simulink model "MIL4L3_SW6_V1_20220211"  (R2018b)
settings: Solver=FixedStepAuto  StartTime=0.0  StopTime=inf  FixedStep=0.001  RelTol=1e-3
PreLoadFcn:
  | A0_MILtest;
undefined symbols (not defined in the file or in its folder): Clb_ICADirect_LaneDisp_StateFive, Clb_ICADirect_LaneDisp_StateFour, Clb_ICADirect_LaneDisp_StateOne, Clb_ICADirect_LaneDisp_StateThree, Clb_ICADirect_LaneDisp_StateTwo, Clb_ICADirect_LaneDisp_StateZero, Clb_ICADirect_LaneDispSW, Clb_ICADirect_TrnLghtsCom_Switch, Clb_ICADirect_TrnLghtsCom_Value, Clb_ICADirect_TrnLghtsCrtl_Inhb, IMAP_Clb_ACU_Driver_Belt, IMAP_Clb_ACU_Driver_Belt_Over, IMAP_Clb_ACU_Passenger_Belt, IMAP_Clb_ACU_Passenger_Belt_Over, IMAP_Clb_ACU_RearLeft_Belt, IMAP_Clb_ACU_RearLeft_Belt_Over, IMAP_Clb_ACU_RearMiddle_Belt, IMAP_Clb_ACU_RearMiddle_Belt_Over, IMAP_Clb_ACU_RearRight_Belt, IMAP_Clb_ACU_RearRight_Belt_Over, IMAP_Clb_AEB_Switch, IMAP_Clb_AEB_Switch_Over, IMAP_Clb_ALC_TLC_Mode, IMAP_Clb_ALC_TLC_Mode_Over, IMAP_Clb_BCM_Battery_Voltage, IMAP_Clb_BCM_Battery_Voltage_Over, IMAP_Clb_BCM_BrakeLamp_State, IMAP_Clb_BCM_BrakeLamp_State_Over, IMAP_Clb_BCM_CHMSL_Status, IMAP_Clb_BCM_CHMSL_Status_Over, IMAP_Clb_BCM_Door_Lock_State, IMAP_Clb_BCM_Door_Lock_State_Over, IMAP_Clb_BCM_FrontWiper_State, IMAP_Clb_BCM_FrontWiper_State_Over, IMAP_Clb_BCM_FrontWiper_Switch, IMAP_Clb_BCM_FrontWiper_Switch_Over, IMAP_Clb_BCM_HazardLamp, IMAP_Clb_BCM_HazardLamp_Over, IMAP_Clb_BCM_HazardLamp_Switch, IMAP_Clb_BCM_HazardLamp_Switch_Over, IMAP_Clb_BCM_HighBeam_State, IMAP_Clb_BCM_HighBeam_State_Over, IMAP_Clb_BCM_Ignition_State, IMAP_Clb_BCM_Ignition_State_Over, IMAP_Clb_BCM_IHBC_Enabled, IMAP_Clb_BCM_IHBC_Enabled_Over, IMAP_Clb_BCM_Left_Light, IMAP_Clb_BCM_Left_Light_Over, IMAP_Clb_BCM_LeftTurn_Switch, IMAP_Clb_BCM_LeftTurn_Switch_Over, IMAP_Clb_BCM_LF_Door_State, IMAP_Clb_BCM_LF_Door_State_Over, IMAP_Clb_BCM_LowBeam_State, IMAP_Clb_BCM_LowBeam_State_Over, IMAP_Clb_BCM_LR_Door_State, IMAP_Clb_BCM_LR_Door_State_Over, IMAP_Clb_BCM_RF_Door_State, IMAP_Clb_BCM_RF_Door_State_Over, IMAP_Clb_BCM_Right_Light, IMAP_Clb_BCM_Right_Light_Over ... (+547)
libraries: CarMaker4SL x2153, simulink x292, dspstat3 x3, canmsglib x2, simulink_extras x1
(part 37 of 52)

== system MIL4L3_SW6_V1_20220211/CarMaker/VehicleControl/OMAP/OMAP1/Runnable_OMAP_10ms_sys/OMAP_Module/Subsystem2 ==
  OMAPve_g_ACCTqReq_1 : Inport
  OMAPve_y_Powertrain_torquewheel_request_1 : Inport  Port=2
  OMAPve_g_TminUp_or_downGear_1 : Inport  Port=3
  OMAPve_y_Function_Acc_status_1 : Inport  Port=4
  Bus Selector5 : BusSelector  OutputSignals=OMAP_clb_ACCTorqueReq_Switch,OMAP_clb_TorqueActivReq_Switch,OMAP_clb_DownorUpGearMinTime_Switch,OMAP_clb_ACCState_Switch
  Constant : Constant  Value=OMAP_clb_ACCTorqueReq
  Constant1 : Constant  Value=OMAP_clb_TorqueActivReq
  Constant2 : Constant  Value=OMAP_clb_DownorUpGearMinTime
  Constant3 : Constant  Value=OMAP_clb_ACCState
  Switch{,1..3} (4 alike) : Switch  Criteria=u2 > Threshold
  Out1 : Outport
  Out2 : Outport  Port=2
  Out3 : Outport  Port=3
  Out4 : Outport  Port=4
  wires:
  Bus Selector5/2 -> Switch1/2  "<OMAP_clb_TorqueActivReq_Switch>"
  Switch2/1 -> Out3/1
  OMAPve_y_Function_Acc_status_1/1 -> Switch3/3
  OMAPve_g_TminUp_or_downGear_1/1 -> Switch2/3
  OMAPve_y_Powertrain_torquewheel_request_1/1 -> Switch1/3
  Bus Selector5/1 -> Switch/2  "<OMAP_clb_ACCTorqueReq_Switch>"
  [ClbBus] -> Bus Selector5/1
  Bus Selector5/3 -> Switch2/2  "<OMAP_clb_DownorUpGearMinTime_Switch>"
  Bus Selector5/4 -> Switch3/2  "<OMAP_clb_ACCState_Switch>"
  OMAPve_g_ACCTqReq_1/1 -> Switch/3
  Switch1/1 -> Out2/1
  Switch3/1 -> Out4/1
  Switch/1 -> Out1/1
  Constant/1 -> Switch/1  "OMAP_clb_ACCTorqueReq"
  Constant1/1 -> Switch1/1  "OMAP_clb_TorqueActivReq"
  Constant2/1 -> Switch2/1  "OMAP_clb_DownorUpGearMinTime"
  Constant3/1 -> Switch3/1  "OMAP_clb_ACCState"

== system MIL4L3_SW6_V1_20220211/CarMaker/VehicleControl/OMAP/OMAP1/Runnable_OMAP_10ms_sys/OMAP_Module/Subsystem3 ==
  OMAPve_g_Deceleration_setpoint_device_1 : Inport
  OMAPve_y_MDD_Decelerationcontrol_request_1 : Inport  Port=2
  OMAPve_y_Prefill_request_1 : Inport  Port=3
  OMAPve_y_ADAS_ESCDriveOff : Inport  Port=4
  OMAPve_y_ADAS_ESCHoldReq : Inport  Port=5
  OMAPve_y_MDD_deceleration_type_1 : Inport  Port=6
  OMAPve_y_AEB_Status_1 : Inport  Port=7
  OMAPve_y_Decel_Request_1 : Inport  Port=8
  OMAPve_y_AEB_Braking_progress_1 : Inport  Port=9
  OMAPve_y_Haptic_Alarm_1 : Inport  Port=10
  OMAPve_y_ADAS_ACCRequestEPB : Inport  Port=11
  Bus Selector5 : BusSelector  OutputSignals=OMAP_clb_DecelerationSet_Switch,OMAP_clb_DeclControlReq_Switch,OMAP_clb_PrefillRequest_Switch,OMAP_clb_ESCDriveOff_Switch,OMAP_clb_ESCHoldReq_Switch,OMAP_clb_DecelerationType_Switch,OMAP_clb_AEBState_Switch,OMAP_clb_BrakeRequest_Switch,OMAP_clb_AEBBrakingProg_Switch,OMAP_clb_HapticAlarmReq_Switch,OMAP_clb_ACCRequestEPB_Switch
  Constant10 : Constant  Value=OMAP_clb_AEBState
  Constant11 : Constant  Value=OMAP_clb_BrakeRequest
  Constant12 : Constant  Value=OMAP_clb_AEBBrakingProg
  Constant13 : Constant  Value=OMAP_clb_HapticAlarmReq
  Constant14 : Constant  Value=OMAP_clb_ACCRequestEPB
  Constant4 : Constant  Value=OMAP_clb_DecelerationSet
  Constant5 : Constant  Value=OMAP_clb_DeclControlReq
  Constant6 : Constant  Value=OMAP_clb_PrefillRequest
  Constant7 : Constant  Value=OMAP_clb_ESCDriveOff
  Constant8 : Constant  Value=OMAP_clb_ESCHoldReq
  Constant9 : Constant  Value=OMAP_clb_DecelerationType
  Switch{,1..10} (11 alike) : Switch  Criteria=u2 > Threshold
  Out1 : Outport
  Out2 : Outport  Port=2
  Out3 : Outport  Port=3
  Out4 : Outport  Port=4
  Out5 : Outport  Port=5
  Out6 : Outport  Port=6
  Out7 : Outport  Port=7
  Out8 : Outport  Port=8
  Out9 : Outport  Port=9
  Out10 : Outport  Port=10
  Out11 : Outport  Port=11
  wires:
  Switch/1 -> Out1/1
  Switch3/1 -> Out4/1
  Switch1/1 -> Out2/1
  OMAPve_g_Deceleration_setpoint_device_1/1 -> Switch/3
  Bus Selector5/4 -> Switch3/2  "<OMAP_clb_ESCDriveOff_Switch>"
  Bus Selector5/3 -> Switch2/2  "<OMAP_clb_PrefillRequest_Switch>"
  [ClbBus] -> Bus Selector5/1
  Bus Selector5/1 -> Switch/2  "<OMAP_clb_DecelerationSet_Switch>"
  OMAPve_y_MDD_Decelerationcontrol_request_1/1 -> Switch1/3
  OMAPve_y_Prefill_request_1/1 -> Switch2/3
  OMAPve_y_ADAS_ESCDriveOff/1 -> Switch3/3
  Switch2/1 -> Out3/1
  Bus Selector5/2 -> Switch1/2  "<OMAP_clb_DeclControlReq_Switch>"
  OMAPve_y_ADAS_ESCHoldReq/1 -> Switch4/3
  Bus Selector5/5 -> Switch4/2  "<OMAP_clb_ESCHoldReq_Switch>"
  Switch4/1 -> Out5/1
  Bus Selector5/6 -> Switch5/2  "<OMAP_clb_DecelerationType_Switch>"
  OMAPve_y_MDD_deceleration_type_1/1 -> Switch5/3
  Switch5/1 -> Out6/1
  Bus Selector5/7 -> Switch6/2  "<OMAP_clb_AEBState_Switch>"
  OMAPve_y_AEB_Status_1/1 -> Switch6/3
  Switch6/1 -> Out7/1
  Bus Selector5/8 -> Switch7/2  "<OMAP_clb_BrakeRequest_Switch>"
  OMAPve_y_Decel_Request_1/1 -> Switch7/3
  Switch7/1 -> Out8/1
  Switch8/1 -> Out9/1
  Bus Selector5/9 -> Switch8/2  "<OMAP_clb_AEBBrakingProg_Switch>"
  OMAPve_y_AEB_Braking_progress_1/1 -> Switch8/3
  Bus Selector5/10 -> Switch9/2  "<OMAP_clb_HapticAlarmReq_Switch>"
  Switch9/1 -> Out10/1
  OMAPve_y_Haptic_Alarm_1/1 -> Switch9/3
  Bus Selector5/11 -> Switch10/2  "<OMAP_clb_ACCRequestEPB_Switch>"
  OMAPve_y_ADAS_ACCRequestEPB/1 -> Switch10/3
  Switch10/1 -> Out11/1
  Constant4/1 -> Switch/1  "OMAP_clb_DecelerationSet"
  Constant5/1 -> Switch1/1  "OMAP_clb_DeclControlReq"
  Constant6/1 -> Switch2/1  "OMAP_clb_PrefillRequest"
  Constant7/1 -> Switch3/1  "OMAP_clb_ESCDriveOff"
  Constant8/1 -> Switch4/1  "OMAP_clb_ESCHoldReq"
  Constant9/1 -> Switch5/1  "OMAP_clb_DecelerationType"
  Constant10/1 -> Switch6/1  "OMAP_clb_AEBState"
  Constant11/1 -> Switch7/1  "OMAP_clb_BrakeRequest"
  Constant12/1 -> Switch8/1  "OMAP_clb_AEBBrakingProg"
  Constant13/1 -> Switch9/1  "OMAP_clb_HapticAlarmReq"
  Constant14/1 -> Switch10/1  "OMAP_clb_ACCRequestEPB"

== system MIL4L3_SW6_V1_20220211/CarMaker/VehicleControl/OMAP/OMAP1/Runnable_OMAP_10ms_sys/OMAP_Module/Subsystem4 ==
  OMAPve_y_General_state_of_LKA_function3F2_2 : Inport
  OMAPve_g_Coefficient_toregulate_EPS_2 : Inport  Port=2
  OMAPve_g_Column_angle_setpoint3F2_2 : Inport  Port=3
  OMAPve_y_Permit_to_know_if_LKA_or_LPA3F2_2 : Inport  Port=4
  OMAPve_y_ADAS_ESAState_2 : Inport  Port=5
  OMAPve_g_ADAS_ESATorqueReq_2 : Inport  Port=6
  OMAPve_y_ADAS_ESARequest_2 : Inport  Port=7
  Bus Selector5 : BusSelector  OutputSignals=OMAP_clb_LKAState_Switch,OMAP_clb_LKATorqFactReq_Switch,OMAP_clb_LKAAngleReq_Switch,OMAP_clb_LKAActivation_Switch,OMAP_clb_ESAState_Switch,OMAP_clb_ESATorqueReq_Switch,OMAP_clb_ESARequest_Switch
  Constant15 : Constant  Value=OMAP_clb_LKAState
  Constant16 : Constant  Value=OMAP_clb_LKATorqFactReq
  Constant17 : Constant  Value=OMAP_clb_LKAAngleReq
  Constant18 : Constant  Value=OMAP_clb_LKAActivation
  Constant19 : Constant  Value=OMAP_clb_ESAState
  Constant20 : Constant  Value=OMAP_clb_ESATorqueReq
  Constant21 : Constant  Value=OMAP_clb_ESARequest
  Switch{,1..6} (7 alike) : Switch  Criteria=u2 > Threshold
  Out1 : Outport
  Out2 : Outport  Port=2
  Out3 : Outport  Port=3
  Out4 : Outport  Port=4
  Out5 : Outport  Port=5
  Out6 : Outport  Port=6
  Out7 : Outport  Port=7
  wires:
  Switch/1 -> Out1/1
  Switch3/1 -> Out4/1
  Switch1/1 -> Out2/1
  OMAPve_y_General_state_of_LKA_function3F2_2/1 -> Switch/3
  Bus Selector5/4 -> Switch3/2  "<OMAP_clb_LKAActivation_Switch>"
  Bus Selector5/3 -> Switch2/2  "<OMAP_clb_LKAAngleReq_Switch>"
  [ClbBus] -> Bus Selector5/1
  Bus Selector5/1 -> Switch/2  "<OMAP_clb_LKAState_Switch>"
  OMAPve_g_Coefficient_toregulate_EPS_2/1 -> Switch1/3
  OMAPve_g_Column_angle_setpoint3F2_2/1 -> Switch2/3
  OMAPve_y_Permit_to_know_if_LKA_or_LPA3F2_2/1 -> Switch3/3
  Switch2/1 -> Out3/1
  Bus Selector5/2 -> Switch1/2  "<OMAP_clb_LKATorqFactReq_Switch>"
  Bus Selector5/5 -> Switch4/2  "<OMAP_clb_ESAState_Switch>"
  OMAPve_y_ADAS_ESAState_2/1 -> Switch4/3
  Switch4/1 -> Out5/1
  Bus Selector5/6 -> Switch5/2  "<OMAP_clb_ESATorqueReq_Switch>"
  OMAPve_g_ADAS_ESATorqueReq_2/1 -> Switch5/3
  Switch5/1 -> Out6/1
  Bus Selector5/7 -> Switch6/2  "<OMAP_clb_ESARequest_Switch>"
  OMAPve_y_ADAS_ESARequest_2/1 -> Switch6/3
  Switch6/1 -> Out7/1
  Constant15/1 -> Switch/1  "OMAP_clb_LKAState"
  Constant16/1 -> Switch1/1  "OMAP_clb_LKATorqFactReq"
  Constant17/1 -> Switch2/1  "OMAP_clb_LKAAngleReq"
  Constant18/1 -> Switch3/1  "OMAP_clb_LKAActivation"
  Constant19/1 -> Switch4/1  "OMAP_clb_ESAState"
  Constant20/1 -> Switch5/1  "OMAP_clb_ESATorqueReq"
  Constant21/1 -> Switch6/1  "OMAP_clb_ESARequest"

== system MIL4L3_SW6_V1_20220211/CarMaker/VehicleControl/OMAP/OMAP1/Runnable_OMAP_10ms_sys/OMAP_Module/Subsystem6 ==
  OMAPve_y_ADAS_ELKPopupMessage_2 : Inport
  OMAPve_y_ADAS_ESAFaultSt_2 : Inport  Port=2
  OMAPve_y_ADAS_HWAMode_2 : Inport  Port=3
  OMAPve_y_ADAS_HWATurnOnIndicator_2 : Inport  Port=4
  OMAPve_y_ADAS_HWAActionSts_2 : Inport  Port=5
  OMAPve_y_ADAS_LightControlValid_2 : Inport  Port=6
  OMAPve_y_ADAS_ISLCState_2 : Inport  Port=7
  OMAPve_y_ADAS_ISLCDriverRemind_2 : Inport  Port=8
  OMAPve_y_ADAS_TurnLightsCommand_2 : Inport  Port=9
  OMAPve_y_ADAS_JAFaultSt_2 : Inport  Port=10
  OMAPve_y_ACC_DesiredHeadway_Display_2 : Inport  Port=11
  OMAPve_y_ACC_DesiredHeadway_Icon_Basic_2 : Inport  Port=12
  OMAPve_y_ACC_Desired_Set_Speed_2 : Inport  Port=13
  OMAPve_y_ACC_Set_Speed_Display_2 : Inport  Port=14
  OMAPve_y_ACC_Vehicle_Icon_Display_2 : Inport  Port=15
  OMAPve_y_RVVACC_Vehiclespeed_request_type_2 : Inport  Port=16
  OMAPve_y_ACC_Pop_Up_Message_2 : Inport  Port=17
  OMAPve_y_AEB_Alert_Req_2 : Inport  Port=18
  OMAPve_y_AEB_Fault_Status_2 : Inport  Port=19
  OMAPve_y_AEB_Switch_Status_2 : Inport  Port=20
  OMAPve_y_AEB_tips_2 : Inport  Port=21
  OMAPve_y_Hands_off_warning_2 : Inport  Port=22
  OMAPve_y_HMI_Popup_Status_2 : Inport  Port=23
  OMAPve_y_Vehicle_Lane_Display_2 : Inport  Port=24
  OMAPve_y_LDW_Flag_2 : Inport  Port=25
  OMAPve_y_LDW_Status_Display_2 : Inport  Port=26
  OMAPve_y_LKA_Mode_from_Camera_2 : Inport  Port=27
  OMAPve_y_LKA_Status_Display_2 : Inport  Port=28
  OMAPve_y_LKA_Switch_State_2 : Inport  Port=29
  OMAPve_y_ADAS_ELKSts_2 : Inport  Port=30
  OMAPve_y_ICA_HMI_Txt_Disp_2 : Inport  Port=31
  OMAPve_y_TJA_status_icon_2 : Inport  Port=32
  Bus Selector5 : BusSelector  OutputSignals=OMAP_clb_ELKPopupMessage_Switch,OMAP_clb_ESAFaultSt_Switch,OMAP_clb_HWAMode_Switch,OMAP_clb_HWATurnOnIdctr_Switch,OMAP_clb_HWAActionSts_Switch,OMAP_clb_LightControlValid_Switch,OMAP_clb_ISLCState_Switch,OMAP_clb_ISLCDriverRemind_Switch,OMAP_clb_TurnLightsCommand_Switch,OMAP_clb_JAFaultSt_Switch,OMAP_clb_ACCHeadwayDisplay_Switch,OMAP_clb_ACCHeadwayIcon_Switch,OMAP_clb_ACCSetSpeed_Switch,OMAP_clb_ACCSetSpeedDis_Switch,OMAP_clb_ACCStatusIconDis_Switch,OMAP_clb_ACC_RVVReqType_Switch,OMAP_clb_ACCMessagePrompt_Switch,OMAP_clb_AEBAlertReq_Switch,OMAP_clb_AEBFaultStatus_Switch,OMAP_clb_AEBSwitchStatus_Switch,OMAP_clb_AEBMassageDisp_Switch,OMAP_clb_Handsoffwarning_Switch,OMAP_clb_HMIPopupMassage_Switch,OMAP_clb_VehicleLaneDisp_Switch,OMAP_clb_LDWWarningSt_Switch,OMAP_clb_LDWStatusDisplay_Switch,OMAP_clb_LKAMode_Switch,OMAP_clb_LKAStatusDisplay_Switch,OMAP_clb_LKASwitchState_Switch,OMAP_clb_ELKSts_Switch,OMAP_clb_ICAMassageDisp_Switch,OMAP_clb_ICAStatusIcon_Switch
  Constant23 : Constant  Value=OMAP_clb_ELKPopupMessage
  Constant24 : Constant  Value=OMAP_clb_ESAFaultSt
  Constant25 : Constant  Value=OMAP_clb_HWAMode
  Constant26 : Constant  Value=OMAP_clb_HWATurnOnIdctr
  Constant27 : Constant  Value=OMAP_clb_HWAActionSts
  Constant28 : Constant  Value=OMAP_clb_LightControlValid
  Constant29 : Constant  Value=OMAP_clb_ISLCState
  Constant30 : Constant  Value=OMAP_clb_ISLCDriverRemind
  Constant31 : Constant  Value=OMAP_clb_TurnLightsCommand
  Constant32 : Constant  Value=OMAP_clb_JAFaultSt
  Constant33 : Constant  Value=OMAP_clb_ACCHeadwayDisplay
  Constant34 : Constant  Value=OMAP_clb_ACCHeadwayIcon
  Constant35 : Constant  Value=OMAP_clb_ACCSetSpeed
  Constant36 : Constant  Value=OMAP_clb_ACCSetSpeedDis
  Constant37 : Constant  Value=OMAP_clb_ACCStatusIconDis
  Constant38 : Constant  Value=OMAP_clb_ACC_RVVReqType
  Constant39 : Constant  Value=OMAP_clb_ACCMessagePrompt
  Constant40 : Constant  Value=OMAP_clb_AEBAlertReq
  Constant41 : Constant  Value=OMAP_clb_AEBFaultStatus
  Constant42 : Constant  Value=OMAP_clb_AEBSwitchStatus
  Constant43 : Constant  Value=OMAP_clb_AEBMassageDisp
  Constant44 : Constant  Value=OMAP_clb_Handsoffwarning
  Constant45 : Constant  Value=OMAP_clb_HMIPopupMassage
  Constant46 : Constant  Value=OMAP_clb_VehicleLaneDisp
  Constant47 : Constant  Value=OMAP_clb_LDWWarningSt
  Constant48 : Constant  Value=OMAP_clb_LDWStatusDisplay
  Constant49 : Constant  Value=OMAP_clb_LKAMode
  Constant50 : Constant  Value=OMAP_clb_LKAStatusDisplay
  Constant51 : Constant  Value=OMAP_clb_LKASwitchState
  Constant52 : Constant  Value=OMAP_clb_ELKSts
  Constant53 : Constant  Value=OMAP_clb_ICAMassageDisp
  Constant54 : Constant  Value=OMAP_clb_ICAStatusIcon
  Switch{,1..31} (32 alike) : Switch  Criteria=u2 > Threshold
  Out1 : Outport
  Out2 : Outport  Port=2
  Out3 : Outport  Port=3
  Out4 : Outport  Port=4
  Out5 : Outport  Port=5
  Out6 : Outport  Port=6
  Out7 : Outport  Port=7
  Out8 : Outport  Port=8
  Out9 : Outport  Port=9
  Out10 : Outport  Port=10
  Out11 : Outport  Port=11
  Out12 : Outport  Port=12
  Out13 : Outport  Port=13
  Out14 : Outport  Port=14
  Out15 : Outport  Port=15
  Out16 : Outport  Port=16
  Out17 : Outport  Port=17
  Out18 : Outport  Port=18
  Out19 : Outport  Port=19
  Out20 : Outport  Port=20
  Out21 : Outport  Port=21
  Out22 : Outport  Port=22
  Out23 : Outport  Port=23
  Out24 : Outport  Port=24
  Out25 : Outport  Port=25
  Out26 : Outport  Port=26
  Out27 : Outport  Port=27
  Out28 : Outport  Port=28
  Out29 : Outport  Port=29
  Out30 : Outport  Port=30
  Out31 : Outport  Port=31
  Out32 : Outport  Port=32
  wires:
  Switch10/1 -> Out11/1
  OMAPve_y_ACC_DesiredHeadway_Display_2/1 -> Switch10/3
  Bus Selector5/11 -> Switch10/2  "<OMAP_clb_ACCHeadwayDisplay_Switch>"
  OMAPve_y_ADAS_JAFaultSt_2/1 -> Switch9/3
  Switch9/1 -> Out10/1
  Bus Selector5/10 -> Switch9/2  "<OMAP_clb_JAFaultSt_Switch>"
  OMAPve_y_ADAS_TurnLightsCommand_2/1 -> Switch8/3
  Bus Selector5/9 -> Switch8/2  "<OMAP_clb_TurnLightsCommand_Switch>"
  Switch8/1 -> Out9/1
  Switch7/1 -> Out8/1
  OMAPve_y_ADAS_ISLCDriverRemind_2/1 -> Switch7/3
  Bus Selector5/8 -> Switch7/2  "<OMAP_clb_ISLCDriverRemind_Switch>"
  Switch6/1 -> Out7/1
  OMAPve_y_ADAS_ISLCState_2/1 -> Switch6/3
  Bus Selector5/7 -> Switch6/2  "<OMAP_clb_ISLCState_Switch>"
  Switch5/1 -> Out6/1
  OMAPve_y_ADAS_LightControlValid_2/1 -> Switch5/3
  Bus Selector5/6 -> Switch5/2  "<OMAP_clb_LightControlValid_Switch>"
  Switch4/1 -> Out5/1
  Bus Selector5/5 -> Switch4/2  "<OMAP_clb_HWAActionSts_Switch>"
  OMAPve_y_ADAS_HWAActionSts_2/1 -> Switch4/3
  Bus Selector5/2 -> Switch1/2  "<OMAP_clb_ESAFaultSt_Switch>"
  Switch2/1 -> Out3/1
  OMAPve_y_ADAS_HWATurnOnIndicator_2/1 -> Switch3/3
  OMAPve_y_ADAS_HWAMode_2/1 -> Switch2/3
  OMAPve_y_ADAS_ESAFaultSt_2/1 -> Switch1/3
  Bus Selector5/1 -> Switch/2  "<OMAP_clb_ELKPopupMessage_Switch>"
  [ClbBus] -> Bus Selector5/1
  Bus Selector5/3 -> Switch2/2  "<OMAP_clb_HWAMode_Switch>"
  Bus Selector5/4 -> Switch3/2  "<OMAP_clb_HWATurnOnIdctr_Switch>"
  OMAPve_y_ADAS_ELKPopupMessage_2/1 -> Switch/3
  Switch1/1 -> Out2/1
  Switch3/1 -> Out4/1
  Switch/1 -> Out1/1
  Bus Selector5/12 -> Switch11/2  "<OMAP_clb_ACCHeadwayIcon_Switch>"
  OMAPve_y_ACC_DesiredHeadway_Icon_Basic_2/1 -> Switch11/3
  Switch11/1 -> Out12/1
  Bus Selector5/13 -> Switch12/2  "<OMAP_clb_ACCSetSpeed_Switch>"
  OMAPve_y_ACC_Desired_Set_Speed_2/1 -> Switch12/3
  Switch12/1 -> Out13/1
  Switch13/1 -> Out14/1
  OMAPve_y_ACC_Set_Speed_Display_2/1 -> Switch13/3
  Bus Selector5/14 -> Switch13/2  "<OMAP_clb_ACCSetSpeedDis_Switch>"
  Bus Selector5/15 -> Switch14/2  "<OMAP_clb_ACCStatusIconDis_Switch>"
  OMAPve_y_ACC_Vehicle_Icon_Display_2/1 -> Switch14/3
  Switch14/1 -> Out15/1
  Switch15/1 -> Out16/1
  OMAPve_y_RVVACC_Vehiclespeed_request_type_2/1 -> Switch15/3
  Bus Selector5/16 -> Switch15/2  "<OMAP_clb_ACC_RVVReqType_Switch>"
  Bus Selector5/17 -> Switch16/2  "<OMAP_clb_ACCMessagePrompt_Switch>"
  OMAPve_y_ACC_Pop_Up_Message_2/1 -> Switch16/3
  Switch16/1 -> Out17/1
  Switch17/1 -> Out18/1
  OMAPve_y_AEB_Alert_Req_2/1 -> Switch17/3
  Bus Selector5/18 -> Switch17/2  "<OMAP_clb_AEBAlertReq_Switch>"
  Bus Selector5/19 -> Switch18/2  "<OMAP_clb_AEBFaultStatus_Switch>"
  OMAPve_y_AEB_Fault_Status_2/1 -> Switch18/3
  Switch18/1 -> Out19/1
  Switch19/1 -> Out20/1
  OMAPve_y_AEB_Switch_Status_2/1 -> Switch19/3
  Bus Selector5/20 -> Switch19/2  "<OMAP_clb_AEBSwitchStatus_Switch>"
  Bus Selector5/21 -> Switch20/2  "<OMAP_clb_AEBMassageDisp_Switch>"
  OMAPve_y_AEB_tips_2/1 -> Switch20/3
  Switch20/1 -> Out21/1
  Switch21/1 -> Out22/1
  OMAPve_y_Hands_off_warning_2/1 -> Switch21/3
  Bus Selector5/22 -> Switch21/2  "<OMAP_clb_Handsoffwarning_Switch>"
  Bus Selector5/23 -> Switch22/2  "<OMAP_clb_HMIPopupMassage_Switch>"
  OMAPve_y_HMI_Popup_Status_2/1 -> Switch22/3
  Switch22/1 -> Out23/1
  Switch23/1 -> Out24/1
  OMAPve_y_Vehicle_Lane_Display_2/1 -> Switch23/3
  Bus Selector5/24 -> Switch23/2  "<OMAP_clb_VehicleLaneDisp_Switch>"
  Bus Selector5/25 -> Switch24/2  "<OMAP_clb_LDWWarningSt_Switch>"
  OMAPve_y_LDW_Flag_2/1 -> Switch24/3
  Switch24/1 -> Out25/1
  Switch25/1 -> Out26/1
  OMAPve_y_LDW_Status_Display_2/1 -> Switch25/3
  Bus Selector5/26 -> Switch25/2  "<OMAP_clb_LDWStatusDisplay_Switch>"
  Bus Selector5/27 -> Switch26/2  "<OMAP_clb_LKAMode_Switch>"
  OMAPve_y_LKA_Mode_from_Camera_2/1 -> Switch26/3
  Switch26/1 -> Out27/1
  Switch27/1 -> Out28/1
  OMAPve_y_LKA_Status_Display_2/1 -> Switch27/3
  Bus Selector5/28 -> Switch27/2  "<OMAP_clb_LKAStatusDisplay_Switch>"
  Bus Selector5/29 -> Switch28/2  "<OMAP_clb_LKASwitchState_Switch>"
  OMAPve_y_LKA_Switch_State_2/1 -> Switch28/3
  Switch28/1 -> Out29/1
  Switch29/1 -> Out30/1
  OMAPve_y_ADAS_ELKSts_2/1 -> Switch29/3
  Bus Selector5/30 -> Switch29/2  "<OMAP_clb_ELKSts_Switch>"
  Bus Selector5/31 -> Switch30/2  "<OMAP_clb_ICAMassageDisp_Switch>"
  OMAPve_y_ICA_HMI_Txt_Disp_2/1 -> Switch30/3
  Switch30/1 -> Out31/1
  Switch31/1 -> Out32/1
  OMAPve_y_TJA_status_icon_2/1 -> Switch31/3
  Bus Selector5/32 -> Switch31/2  "<OMAP_clb_ICAStatusIcon_Switch>"
  Constant23/1 -> Switch/1  "OMAP_clb_ELKPopupMessage"
  Constant24/1 -> Switch1/1  "OMAP_clb_ESAFaultSt"
  Constant25/1 -> Switch2/1  "OMAP_clb_HWAMode"
  Constant26/1 -> Switch3/1  "OMAP_clb_HWATurnOnIdctr"
  Constant27/1 -> Switch4/1  "OMAP_clb_HWAActionSts"
  Constant28/1 -> Switch5/1  "OMAP_clb_LightControlValid"
  Constant29/1 -> Switch6/1  "OMAP_clb_ISLCState"
  Constant30/1 -> Switch7/1  "OMAP_clb_ISLCDriverRemind"
  Constant31/1 -> Switch8/1  "OMAP_clb_TurnLightsCommand"
  Constant32/1 -> Switch9/1  "OMAP_clb_JAFaultSt"
  Constant33/1 -> Switch10/1  "OMAP_clb_ACCHeadwayDisplay"
  Constant34/1 -> Switch11/1  "OMAP_clb_ACCHeadwayIcon"
  Constant35/1 -> Switch12/1  "OMAP_clb_ACCSetSpeed"
  Constant36/1 -> Switch13/1  "OMAP_clb_ACCSetSpeedDis"
  Constant37/1 -> Switch14/1  "OMAP_clb_ACCStatusIconDis"
  Constant38/1 -> Switch15/1  "OMAP_clb_ACC_RVVReqType"
  Constant39/1 -> Switch16/1  "OMAP_clb_ACCMessagePrompt"
  Constant40/1 -> Switch17/1  "OMAP_clb_AEBAlertReq"
  Constant41/1 -> Switch18/1  "OMAP_clb_AEBFaultStatus"
  Constant42/1 -> Switch19/1  "OMAP_clb_AEBSwitchStatus"
  Constant43/1 -> Switch20/1  "OMAP_clb_AEBMassageDisp"
  Constant44/1 -> Switch21/1  "OMAP_clb_Handsoffwarning"
  Constant45/1 -> Switch22/1  "OMAP_clb_HMIPopupMassage"
  Constant46/1 -> Switch23/1  "OMAP_clb_VehicleLaneDisp"
  Constant47/1 -> Switch24/1  "OMAP_clb_LDWWarningSt"
  Constant48/1 -> Switch25/1  "OMAP_clb_LDWStatusDisplay"
  Constant49/1 -> Switch26/1  "OMAP_clb_LKAMode"
  Constant50/1 -> Switch27/1  "OMAP_clb_LKAStatusDisplay"
  Constant51/1 -> Switch28/1  "OMAP_clb_LKASwitchState"
  Constant52/1 -> Switch29/1  "OMAP_clb_ELKSts"
  Constant53/1 -> Switch30/1  "OMAP_clb_ICAMassageDisp"
  Constant54/1 -> Switch31/1  "OMAP_clb_ICAStatusIcon"

== system MIL4L3_SW6_V1_20220211/CarMaker/VehicleControl/OMAP/OMAP1/Runnable_OMAP_10ms_sys/OMAP_Module/Subsystem7 ==
  OMAPve_y_ADAS_LCAStatusDisplay1 : Inport
  OMAPve_y_ADAS_LCAPopupMessage1 : Inport  Port=2
  OMAPve_y_ADAS_State1 : Inport  Port=3
  Bus Selector5 : BusSelector  OutputSignals=OMAP_clb_LCAStatusDisplay_Switch,OMAP_clb_LCAPopupMessage_Switch,OMAP_clb_ADAS_State_Switch
  Constant55 : Constant  Value=OMAP_clb_LCAStatusDisplay
  Constant56 : Constant  Value=OMAP_clb_LCAPopupMessage
  Constant57 : Constant  Value=OMAP_clb_ADAS_State
  Switch : Switch  Criteria=u2 > Threshold
  Switch1 : Switch  Criteria=u2 > Threshold
  Switch2 : Switch  Criteria=u2 > Threshold
  Out1 : Outport
  Out2 : Outport  Port=2
  Out3 : Outport  Port=3
  wires:
  Switch/1 -> Out1/1
  Switch1/1 -> Out2/1
  OMAPve_y_ADAS_LCAStatusDisplay1/1 -> Switch/3
  Bus Selector5/3 -> Switch2/2  "<OMAP_clb_ADAS_State_Switch>"
  [ClbBus] -> Bus Selector5/1
  Bus Selector5/1 -> Switch/2  "<OMAP_clb_LCAStatusDisplay_Switch>"
  OMAPve_y_ADAS_LCAPopupMessage1/1 -> Switch1/3
  OMAPve_y_ADAS_State1/1 -> Switch2/3
  Switch2/1 -> Out3/1
  Bus Selector5/2 -> Switch1/2  "<OMAP_clb_LCAPopupMessage_Switch>"
  Constant55/1 -> Switch/1  "OMAP_clb_LCAStatusDisplay"
  Constant56/1 -> Switch1/1  "OMAP_clb_LCAPopupMessage"
  Constant57/1 -> Switch2/1  "OMAP_clb_ADAS_State"

== system MIL4L3_SW6_V1_20220211/CarMaker/VehicleControl/OMAP/OMAP1/Runnable_OMAP_10ms_sys/OMAP_Module/Subsystem8 ==
  OMAPve_y_TYPE_RAPPORT_2 : Inport
  Bus Selector5 : BusSelector  OutputSignals=OMAP_clb_UpDownGearChange_Switch
  Constant22 : Constant  Value=OMAP_clb_UpDownGearChange
  Switch : Switch  Criteria=u2 > Threshold
  Out1 : Outport
  wires:
  Bus Selector5/1 -> Switch/2  "<OMAP_clb_UpDownGearChange_Switch>"
  [ClbBus] -> Bus Selector5/1
  OMAPve_y_TYPE_RAPPORT_2/1 -> Switch/3
  Switch/1 -> Out1/1
  Constant22/1 -> Switch/1  "OMAP_clb_UpDownGearChange"

== system MIL4L3_SW6_V1_20220211/CarMaker/VehicleControl/Function/LKA/LKAS1/LL/Human Machine Interface (HMI)/Subsystem ==
  LDW_STATE : Inport
  LKA_STATE : Inport  Port=2
  EPSInfo : Inport  Port=3
  SampleTime : Inport  Port=4
  HandsOff_Text : Inport  Port=5
  HandsOff_Warn : Inport  Port=6
  Abs : Abs
  Bus Selector2 : BusSelector  OutputSignals=EPS_LKA_State,EPS_SW_Trq
  Compare{1..2,4,7} (4 alike) : simulink/Logic and Bit Operations/Compare To Constant  relop===  const=3  OutDataTypeStr=boolean
  Compare3 : simulink/Logic and Bit Operations/Compare To Constant  relop===  const=1  OutDataTypeStr=boolean
  Compare5 : simulink/Logic and Bit Operations/Compare To Constant  relop===  const=4  OutDataTypeStr=boolean
  Compare6 : simulink/Logic and Bit Operations/Compare To Constant  relop===  const=5  OutDataTypeStr=boolean
  Compare8 : simulink/Logic and Bit Operations/Compare To Constant  relop===  const=4  OutDataTypeStr=boolean
  Compare9 : simulink/Logic and Bit Operations/Compare To Constant  relop===  const=5  OutDataTypeStr=boolean
  Constant : Constant  Value=0.25  OutDataTypeStr=single
  Constant1 : Constant  Value=0.5  OutDataTypeStr=single
  Logical Operator1 : Logic  Operator=OR  AllPortsSameDT=off  OutDataTypeStr=boolean
  Logical Operator2 : Logic  Inputs=3  AllPortsSameDT=off  OutDataTypeStr=boolean
  Logical Operator3 : Logic  Operator=OR  Inputs=6  AllPortsSameDT=off  OutDataTypeStr=boolean
  Relational Operator : RelationalOperator  Operator=<=  OutDataTypeStr=boolean  RndMeth=Nearest
  Sum Condition1 : Subsystem  TreatAsAtomicUnit=on
  Sum Condition2 : Subsystem  TreatAsAtomicUnit=on
  Switch : Switch  Criteria=u2 > Threshold
  HandsOff2_Warn : Outport
  HandsOff1_Text : Outport  Port=2
  wires:
  Sum Condition1/1(Out) -> HandsOff1_Text/1
  Bus Selector2/1 -> Compare3/1, Compare2/1, Compare1/1  "<EPS_LKA_State>"
  Constant/1 -> Switch/3
  EPSInfo/1 -> Bus Selector2/1
  Switch/1 -> Relational Operator/2
  Compare1/1 -> Switch/2
  Bus Selector2/2 -> Abs/1  "<EPS_SW_Trq>"
  Logical Operator2/1 -> Sum Condition1/Enable, Sum Condition2/Enable
  Logical Operator3/1 -> Logical Operator2/1
  Constant1/1 -> Switch/1
  Relational Operator/1 -> Logical Operator2/3
  Sum Condition2/1(Out) -> HandsOff2_Warn/1
  LDW_STATE/1 -> Compare4/1, Compare6/1, Compare5/1
  Compare4/1 -> Logical Operator3/3
  Compare5/1 -> Logical Operator3/2
  Compare6/1 -> Logical Operator3/1
  Abs/1 -> Relational Operator/1
  LKA_STATE/1 -> Compare9/1, Compare8/1, Compare7/1
  Compare9/1 -> Logical Operator3/4
  Compare8/1 -> Logical Operator3/5
  Compare7/1 -> Logical Operator3/6
  Compare2/1 -> Logical Operator1/1
  Compare3/1 -> Logical Operator1/2
  Logical Operator1/1 -> Logical Operator2/2
  SampleTime/1 -> Sum Condition2/1(SampleTime), Sum Condition1/1(SampleTime)
  HandsOff_Text/1 -> Sum Condition1/2(Sum)
  HandsOff_Warn/1 -> Sum Condition2/2(Sum)

== system MIL4L3_SW6_V1_20220211/CarMaker/VehicleControl/Function/LKA/LKAS1/LL/LL Inputs Mapping/bsBCMInfo ==
  bsBCMInfoIn : Inport
  Bus Creator1 : BusCreator  Inputs=3
  Bus Selector1 : BusSelector  OutputSignals=BCM_Double_Light,BCM_Left_Light,BCM_Right_Light,BCM_LeftTurn_Switch,BCM_RightTurn_Switch
  Compare To Constant : simulink/Logic and Bit Operations/Compare To Constant  relop===  const=1  OutDataTypeStr=boolean
  Compare To Constant1 : simulink/Logic and Bit Operations/Compare To Constant  relop===  const=1  OutDataTypeStr=boolean
  Logical Operator : Logic  Operator=OR  AllPortsSameDT=off  OutDataTypeStr=boolean
  Logical Operator1 : Logic  Operator=OR  AllPortsSameDT=off  OutDataTypeStr=boolean
  bsBCMInfoOut : Outport
  wires:
  Bus Selector1/3 -> Logical Operator1/1  "<BCM_Right_Light>"
  Bus Selector1/2 -> Logical Operator/1  "<BCM_Left_Light>"
  Bus Creator1/1 -> bsBCMInfoOut/1
  Bus Selector1/1 -> Bus Creator1/1  "<BCM_Double_Light>"
  bsBCMInfoIn/1 -> Bus Selector1/1
  Bus Selector1/4 -> Compare To Constant/1  "<BCM_LeftTurn_Switch>"
  Bus Selector1/5 -> Compare To Constant1/1  "<BCM_RightTurn_Switch>"
  Compare To Constant/1 -> Logical Operator/2
  Compare To Constant1/1 -> Logical Operator1/2
  Logical Operator/1 -> Bus Creator1/2  "BCM_Left_Light"
  Logical Operator1/1 -> Bus Creator1/3  "BCM_Right_Light"

== system MIL4L3_SW6_V1_20220211/CarMaker/VehicleControl/Function/LKA/LKAS1/LL/LL Inputs Mapping/bsEPSInfo ==
  bsEPSInfoIn : Inport
  Bus Creator4 : BusCreator  Inputs=11
  Bus Selector1 : BusSelector  OutputSignals=EPS_LKA_State,EPS_SW_Trq,EPS_Trq_State,SAS_Clb_State,SAS_Trim_State,SWS_Failure_Status,EPS_TrqLim_State,EPS_LKA_Current,EPS_SWHold_State,EPS_Driver_Override,EPS_ESA_State
  bsEPSInfoOut : Outport
  wires:
  Bus Selector1/9 -> Bus Creator4/9  "<EPS_SWHold_State>"
  Bus Selector1/8 -> Bus Creator4/8  "<EPS_LKA_Current>"
  Bus Selector1/7 -> Bus Creator4/7  "<EPS_TrqLim_State>"
  Bus Selector1/5 -> Bus Creator4/5  "<SAS_Trim_State>"
  Bus Selector1/4 -> Bus Creator4/4  "<SAS_Clb_State>"
  Bus Selector1/3 -> Bus Creator4/3  "<EPS_Trq_State>"
  Bus Creator4/1 -> bsEPSInfoOut/1
  Bus Selector1/1 -> Bus Creator4/1  "<EPS_LKA_State>"
  Bus Selector1/2 -> Bus Creator4/2  "<EPS_SW_Trq>"
  bsEPSInfoIn/1 -> Bus Selector1/1
  Bus Selector1/6 -> Bus Creator4/6  "<SWS_Failure_Status>"
  Bus Selector1/10 -> Bus Creator4/10  "<EPS_Driver_Override>"
  Bus Selector1/11 -> Bus Creator4/11  "<EPS_ESA_State>"

== system MIL4L3_SW6_V1_20220211/CarMaker/VehicleControl/Function/LKA/LKAS1/LL/LL Inputs Mapping/bsLaneInfo ==
  bsLLClb : Inport
  bsLaneInfoIn : Inport  Port=2
  Bus Creator : BusCreator  Inputs=5
  Bus Selector1 : BusSelector  OutputSignals=bsFusL0Info,bsFusR0Info,bsFusL1Info,bsFusR1Info,Fusion_AdditionalInf
  LaneSelect : Subsystem
  "LanesReconstruct " : Subsystem
  bsLaneInfoOut : Outport
  wires:
  Bus Creator/1 -> bsLaneInfoOut/1
  Bus Selector1/4 -> LaneSelect/4(bsFusR1Info)  "<bsFusR1Info>"
  Bus Selector1/3 -> LaneSelect/3(bsFusL1Info)  "<bsFusL1Info>"
  Bus Selector1/2 -> LaneSelect/2(bsFusR0Info)  "<bsFusR0Info>"
  Bus Selector1/1 -> LaneSelect/1(bsFusL0Info)  "<bsFusL0Info>"
  LaneSelect/4(bsR1Info) -> "LanesReconstruct "/5(bsR1Info)
  LaneSelect/3(bsL1Info) -> "LanesReconstruct "/4(bsL1Info)
  LaneSelect/2(bsR0Info) -> "LanesReconstruct "/3(bsR0Info)
  LaneSelect/1(bsL0Info) -> "LanesReconstruct "/2(bsL0Info)
  "LanesReconstruct "/4(bsR1InfoR) -> Bus Creator/4  "bsR1Info"
  "LanesReconstruct "/3(bsL1InfoR) -> Bus Creator/3  "bsL1Info"
  "LanesReconstruct "/2(bsR0InfoR) -> Bus Creator/2  "bsR0Info"
  "LanesReconstruct "/1(bsL0InfoR) -> Bus Creator/1  "bsL0Info"
  Bus Selector1/5 -> Bus Creator/5  "<Fusion_AdditionalInf>"
  bsLaneInfoIn/1 -> Bus Selector1/1
  bsLLClb/1 -> "LanesReconstruct "/1(bsLLClb)

== system MIL4L3_SW6_V1_20220211/CarMaker/VehicleControl/Function/LKA/LKAS1/LL/LL Inputs Mapping/bsMP5Info ==
  note: LkaFcnConf
      | 0: OFF
      | 1: LDW-声音
      | 2: LDW-振动
      | 3: LDW-声音+振动
      | 4: LKA-声音
      | 5: LKA-振动
      | 6: LKA-声音+振动
      | 7: LDW-声音-ICA
      | 8: LDW-振动-ICA
      | 9: LDW-声音+振动-ICA
      | 10: LKA-声音-ICA
      | 11: LKA-振动-ICA
      | 12: LKA-声音+振动-ICA
  bsMP5InfoIn : Inport
  Add : Sum
  Add1 : Sum  Inputs=+-  OutMin=0  OutMax=12
  Bus Creator : BusCreator  Inputs=5
  Bus Selector1 : BusSelector  OutputSignals=LkaFcnConf,LKA_Main_Switch,LKA_Mode,LDW_Warn_Mode,APA_AutoPark_WorkSt,MP5_Work_State
  Constant1 : Constant  OutDataTypeStr=uint8
  Constant2 : Constant  Value=6  OutDataTypeStr=uint8
  Constant3 : Constant  OutDataTypeStr=uint8
  Constant4 : Constant  Value=0  OutDataTypeStr=uint8
  Constant5 : Constant  Value=3  OutDataTypeStr=uint8
  Constant6 : Constant  OutDataTypeStr=uint8
  Constant7 : Constant  Value=3  OutDataTypeStr=uint8
  Divide : Product  Inputs=**  OutDataTypeStr=uint8
  Divide1 : Product  Inputs=*/
  Logical Operator : Logic  Operator=OR  AllPortsSameDT=off  OutDataTypeStr=boolean
  Max : MinMax  Function=max  Inputs=2
  Max1 : MinMax  Function=max  Inputs=2
  Mod : Math  Operator=mod  SaturateOnIntegerOverflow=on
  Mod1 : Math  Operator=mod  SaturateOnIntegerOverflow=on
  Saturation : Saturate  UpperLimit=12  LowerLimit=0
  Saturation1 : Saturate  UpperLimit=12  LowerLimit=1
  Switch : Switch  Criteria=u2 > Threshold
  bsMP5InfoOut : Outport
  wires:
  bsMP5InfoIn/1 -> Bus Selector1/1
  Divide/1 -> Bus Creator/2  "LKA_Mode"
  Bus Selector1/2 -> Logical Operator/2  "<LKA_Main_Switch>"
  Add/1 -> Divide/2
  Bus Selector1/3 -> Max/2  "<LKA_Mode>"
  Constant6/1 -> Add/2
  Bus Selector1/1 -> Switch/2, Saturation1/1  "<LkaFcnConf>"
  Constant1/1 -> Add1/2
  Add1/1 -> Saturation/1
  Constant2/1 -> Mod/2
  Constant3/1 -> Switch/1
  Constant4/1 -> Switch/3
  Switch/1 -> Logical Operator/1
  Logical Operator/1 -> Divide/1, Bus Creator/1  "LKA_Main_Switch"
  Bus Selector1/5 -> Bus Creator/4  "<APA_AutoPark_WorkSt>"
  Bus Selector1/6 -> Bus Creator/5  "<MP5_Work_State>"
  Bus Creator/1 -> bsMP5InfoOut/1
  Saturation/1 -> Mod1/1, Mod/1
  Mod/1 -> Divide1/1
  Constant5/1 -> Divide1/2
  Divide1/1 -> Max/1
  Max/1 -> Add/1
  Constant7/1 -> Mod1/2
  Mod1/1 -> Max1/1
  Bus Selector1/4 -> Max1/2  "<LDW_Warn_Mode>"
  Max1/1 -> Bus Creator/3  "LDW_Warn_Mode"
  Saturation1/1 -> Add1/1

== system MIL4L3_SW6_V1_20220211/CarMaker/VehicleControl/Function/LKA/LKAS1/LL/LL Inputs Mapping/bsPTState ==
  bsPTStateIn : Inport
  Bus Creator3 : BusCreator  Inputs=3
  Bus Selector1 : BusSelector  OutputSignals=AccPedal_Pos,TCU_ActualGear,TCU_Available
  Constant1 : Constant  Value=0  OutDataTypeStr=uint8
  Constant3 : Constant  Value=3  OutDataTypeStr=uint8
  Multiport Switch : MultiPortSwitch  DataPortOrder=Zero-based contiguous  Inputs=11  zeroidx=on
  bsPTStateOut : Outport
  wires:
  Bus Creator3/1 -> bsPTStateOut/1
  Bus Selector1/1 -> Bus Creator3/1  "<AccPedal_Pos>"
  bsPTStateIn/1 -> Bus Selector1/1
  Multiport Switch/1 -> Bus Creator3/2  "TCU_ActualGear"
  Constant3/1 -> Multiport Switch/11, Multiport Switch/10, Multiport Switch/9, Multiport Switch/6, Multiport Switch/5, Multiport Switch/4, Multiport Switch/3
  Bus Selector1/2 -> Multiport Switch/1  "<TCU_ActualGear>"
  Constant1/1 -> Multiport Switch/12, Multiport Switch/8, Multiport Switch/7, Multiport Switch/2
  Bus Selector1/3 -> Bus Creator3/3  "<TCU_Available>"

== system MIL4L3_SW6_V1_20220211/CarMaker/VehicleControl/Function/LKA/LKAS1/LL/LL Inputs Mapping/bsSWAInfo ==
  bsSWAInfoIn : Inport
  Bus Creator : BusCreator  Inputs=4
  Bus Selector1 : BusSelector  OutputSignals=EPS_SteeringAngle_Flag,EPS_SteeringAngle,SW_Angle,SW_Angle_Speed
  bsSWAInfoOut : Outport
  wires:
  Bus Creator/1 -> bsSWAInfoOut/1
  Bus Selector1/4 -> Bus Creator/4  "<SW_Angle_Speed>"
  Bus Selector1/3 -> Bus Creator/3  "<SW_Angle>"
  bsSWAInfoIn/1 -> Bus Selector1/1
  Bus Selector1/2 -> Bus Creator/2  "<EPS_SteeringAngle>"
  Bus Selector1/1 -> Bus Creator/1  "<EPS_SteeringAngle_Flag>"

== system MIL4L3_SW6_V1_20220211/CarMaker/VehicleControl/Function/LKA/LKAS1/LL/LL Inputs Mapping/bsVehMovInfo ==
  bsVehMovInfoIn : Inport
  Bus Creator : BusCreator  Inputs=10
  Bus Selector2 : BusSelector  OutputSignals=ESC_LatAcc,ESC_LatAcc_Valid,ESC_YawRate,ESC_YawRate_Valid,ESC_UnYawRate,ESC_VehSpd,ESC_LonAcc,ESC_LonAcc_Valid,ESC_Brake_Press,ESC_VehSpd_Valid
  bsVehMovInfoOut : Outport
  wires:
  Bus Creator/1 -> bsVehMovInfoOut/1
  Bus Selector2/10 -> Bus Creator/10  "<ESC_VehSpd_Valid>"
  Bus Selector2/9 -> Bus Creator/9  "<ESC_Brake_Press>"
  Bus Selector2/8 -> Bus Creator/8  "<ESC_LonAcc_Valid>"
  Bus Selector2/7 -> Bus Creator/7  "<ESC_LonAcc>"
  Bus Selector2/6 -> Bus Creator/6  "<ESC_VehSpd>"
  Bus Selector2/5 -> Bus Creator/5  "<ESC_UnYawRate>"
  Bus Selector2/4 -> Bus Creator/4  "<ESC_YawRate_Valid>"
  Bus Selector2/3 -> Bus Creator/3  "<ESC_YawRate>"
  Bus Selector2/2 -> Bus Creator/2  "<ESC_LatAcc_Valid>"
  Bus Selector2/1 -> Bus Creator/1  "<ESC_LatAcc>"
  bsVehMovInfoIn/1 -> Bus Selector2/1

== system MIL4L3_SW6_V1_20220211/CarMaker/VehicleControl/Function/LKA/LKAS1/LL/LLOn/LDW ==
  LDW_bsLKAInfoSyn : Inport
  LDW_bsLDWClb : Inport  Port=2
  Enable : EnablePort  StatesWhenEnabling=reset  ShowOutputPort=on
      settings: AttributesFormatString=states = %<StatesWhenEnabling>
  Bus Selector : BusSelector  OutputSignals=bsHdAgInfo.phiHdAg_Lft,bsHdAgInfo.phiHdAg_Rgt
  Bus Selector1 : BusSelector  OutputSignals=bsLDWClb.LL_LDWS_SUPPRESS_HEADING,bsConstantClb.LKA_SampleTime
  Cast : DataTypeConversion  OutDataTypeStr=uint8
  Heading Angle Detection (HdAgDet) : Subsystem  Description=|
      | Block Name: Heading Angle Detection
      | Ab.: HdAgDet
      | No.: 1.3.1.0
      | Rev: 0.0.1
      | Update Date: 19-3-26
  Logical Operator : Logic  Operator=NOT  AllPortsSameDT=off  OutDataTypeStr=boolean
  Product : Product  OutDataTypeStr=uint8
  LDW_Flag : Outport  OutputWhenDisabled=reset  InitialOutput=0
      settings: AttributesFormatString=%<OutputWhenDisabled> = %<InitialOutput>
  wires:
  Logical Operator/1 -> Cast/1
  Cast/1 -> Product/2
  Bus Selector1/2 -> Heading Angle Detection (HdAgDet)/5(SampleTime)  "<LKA_SampleTime>"
  Product/1 -> LDW_Flag/1
  Heading Angle Detection (HdAgDet)/1(HdAgDet_stHdAgDetFlg) -> Logical Operator/1
  LDW_bsLKAInfoSyn/1 -> Bus Selector/1
  Enable/1 -> Heading Angle Detection (HdAgDet)/1(HdAgDet_stLDWActvFlg), Product/1
  Bus Selector/1 -> Heading Angle Detection (HdAgDet)/2(HdAgDet_phiHdAgLft)  "<phiHdAg_Lft>"
  Bus Selector/2 -> Heading Angle Detection (HdAgDet)/3(HdAgDet_phiHdAgRgt)  "<phiHdAg_Rgt>"
  LDW_bsLDWClb/1 -> Bus Selector1/1
  Bus Selector1/1 -> Heading Angle Detection (HdAgDet)/4(HdAgDet_phiHdAgThres_C)  "<LL_LDWS_SUPPRESS_HEADING>"

== system MIL4L3_SW6_V1_20220211/CarMaker/VehicleControl/Function/LKA/LKAS1/LL/LLOn/LKA ==
  LKA_bsInInfoSyn : Inport
  LKA_bsLKAInPInfo : Inport  Port=2
  LKA_bsLKAClb : Inport  Port=3
  Enable : EnablePort  StatesWhenEnabling=reset  ShowOutputPort=on
      settings: AttributesFormatString=states = %<StatesWhenEnabling>
  Bus Selector : BusSelector  OutputSignals=bsConstantClb.LKA_SampleTime
  Cast To Single : DataTypeConversion  OutDataTypeStr=uint8
  Driver Torque Addition (DTA) : Subsystem
  LKA Exit Processing (LKAExPrcs) : Subsystem  Description=|
      | Block Name: LKA Exit Processing 
      | Ab.: LKAExPrcs
      | No.: 1.2.2.0
      | Rev: 0.0.1
      | Update Date: 19-5-13
  "LKA Motion Planning (LKAMP) " : Subsystem  Description=|
      | Block Name: LKA Motion Planning
      | Ab.: LKAMP
      | No.: 1.2.3.0
      | Rev: 0.0.1
      | Update Date: 19-5-13
  LKA SWA Limit (LKASWALim) : Subsystem  Description=|
      | Block Name: LKA SWA Synthesis
      | Ab.: LKASWASyn
      | No.: 1.2.6.0
      | Rev: 0.0.1
      | Update Date: 19-5-13
  LKA_Mon : Subsystem
  Lane Following (LF) : Subsystem  Description=|
      | Block Name: Lane Following
      | Ab.: LF
      | No.: 02
      | Rev: 00.00.01
      | Update Date: 19-3-28
  Plan To LaneFollowing (PTLF) : Subsystem
  LKA_ExitFlg : Outport  OutputWhenDisabled=reset  InitialOutput=0
      settings: AttributesFormatString=%<OutputWhenDisabled> = %<InitialOutput>
  LKA_phiSWACmd : Outport  Port=2  OutputWhenDisabled=reset  InitialOutput=0
      settings: AttributesFormatString=%<OutputWhenDisabled> = %<InitialOutput>
  LKA_M : Outport  Port=3  OutputWhenDisabled=reset  InitialOutput=0
      settings: AttributesFormatString=%<OutputWhenDisabled> = %<InitialOutput>
  LKAMon : Outport  Port=4  OutputWhenDisabled=reset  InitialOutput=0
      settings: AttributesFormatString=%<OutputWhenDisabled> = %<InitialOutput>
  tag scope: ActFlg=global, Ff=global, LKA_ExitFlg_Mon=global, LKA_SampleTime=global, PT1=global
  wires:
  Cast To Single/1 -> [ActFlg]  "ActFlg"
  Plan To LaneFollowing (PTLF)/1(SWACmd) -> LKA SWA Limit (LKASWALim)/1(LKASWALim_phiTFCSWACmd)  "PTLFSWACmd"
  Enable/1 -> Cast To Single/1
  LKA SWA Limit (LKASWALim)/1(LKASWALim_phiSWACmd) -> LKA_phiSWACmd/1  "phiSWACmd"
  LKA Exit Processing (LKAExPrcs)/1(LKAExPrcs_stExFlg) -> LKA_ExitFlg/1, [LKA_ExitFlg_Mon]
  [Ff] -> Plan To LaneFollowing (PTLF)/5(Ff)
  [P] -> Plan To LaneFollowing (PTLF)/6(P)
  [I] -> Plan To LaneFollowing (PTLF)/7(I)
  [D] -> Plan To LaneFollowing (PTLF)/8(D)
  Driver Torque Addition (DTA)/1(DTA_phiDTASWACmd) -> [DT]  "DT"
  [DT] -> Plan To LaneFollowing (PTLF)/4(DrvTrq)
  [Plan] -> Plan To LaneFollowing (PTLF)/2(Plan)
  [PT1] -> Plan To LaneFollowing (PTLF)/3(T1)
  [PT1] -> LKA Exit Processing (LKAExPrcs)/3(LKAExPrcs_PlanT1)
  [ActFlg] -> "LKA Motion Planning (LKAMP) "/3(LKAMP_stLKAActvFlg)
  LKA_bsLKAInPInfo/1 -> [LKAInPInfo]
  [LKAInPInfo] -> "LKA Motion Planning (LKAMP) "/4(LKAMP_bsLKAInPInfo)
  [LKAInPInfo] -> LKA Exit Processing (LKAExPrcs)/1(LKAExPrcs_bsLKAInPInfo)
  [LKAInPInfo] -> Plan To LaneFollowing (PTLF)/1(InP)
  LKA_bsLKAClb/1 -> Bus Selector/1, [LKA_bsLLClb]
  [LKAInPInfo] -> LKA SWA Limit (LKASWALim)/3(LKASWALim_bsLKAInPInfo)
  [LKA_bsLLClb] -> LKA Exit Processing (LKAExPrcs)/2(LKAExPrcs_bsLKAClb)
  [LKA_bsLLClb] -> Driver Torque Addition (DTA)/2(DTA_bsLFClb)
  [LKA_bsLLClb] -> Lane Following (LF)/3(LF_bsLFClb)
  [LKA_bsLLClb] -> LKA SWA Limit (LKASWALim)/4(LKASWALim_bsLKAClb)
  LKA_bsInInfoSyn/1 -> [LKA_bsInInfoSyn]
  [LKA_bsInInfoSyn] -> "LKA Motion Planning (LKAMP) "/1(LKAMP_bsInInfoSyn)
  [LKA_bsInInfoSyn] -> Driver Torque Addition (DTA)/1(DTA_bsInInfoSyn)
  [LKA_bsInInfoSyn] -> Lane Following (LF)/1(LF_bsInInfoSyn)
  [Ff] -> LKA SWA Limit (LKASWALim)/2(LKASWALim_Ff)
  [LKAInPInfo] -> Lane Following (LF)/2(LF_bsLKAInPInfo)
  Driver Torque Addition (DTA)/2(DTA_M) -> LKA_M/1
  Lane Following (LF)/3(LF_phiIntegSWACmd) -> [I]
  Lane Following (LF)/1(LF_phiFfLFSWACmd) -> [Ff]
  Lane Following (LF)/2(LF_phiPropSWACmd) -> [P]
  Lane Following (LF)/4(LF_phiDiffSWACmd) -> [D]
  "LKA Motion Planning (LKAMP) "/1(LKAMP_phiSWACmd) -> [Plan]  "PlanSWACmd"
  "LKA Motion Planning (LKAMP) "/3(LKAMP_tiT2) -> ?  "PlanT2"
  "LKA Motion Planning (LKAMP) "/2(LKAMP_tiT1) -> [PT1]  "PlanT1"
  LKA_Mon/1(LKAMon) -> LKAMon/1
  [LKA_bsLLClb] -> "LKA Motion Planning (LKAMP) "/5(LKAMP_bsLLClb)
  Bus Selector/1 -> [LKA_SampleTime]  "<LKA_SampleTime>"
  [Ff] -> "LKA Motion Planning (LKAMP) "/2(In2)

== system MIL4L3_SW6_V1_20220211/CarMaker/VehicleControl/Function/LKA/LKAS1/LL/LLOn/LKA Input Processing (LKAInP) ==
  LKAInP_bsInInfoSyn : Inport
  LKAInP_bsLLClb : Inport  Port=2
  In3 : Inport  Port=3
  Bus Creator2 : BusCreator  Inputs=10
  Curvature Calculation (Crvt) : Subsystem
  Delay : Delay  DelayLength=1
  Deviation Calculation (Dvt) : Subsystem
  Heading Angle Calculation (HdAg) : Subsystem
  Lane Width Calculation (LW) : Subsystem
  Previewed Curvature Calculation (PrCrvt) : Subsystem
  Previewed Deviation Calculation (PrDvt) : Subsystem
  Previewed Heading Angle Calculation (PrHdAg) : Subsystem
  Steering Wheel Position Calculation (SWAPosCal) : Subsystem
  TTLC Calculation (TTLCCalc) : Subsystem  Description=|
      | Block Name: TTLC Calculation
      | Ab.: TTLCCalc
      | No.: 1.1.1.1
      | Rev: 0.0.1
      | Update Date: 19-3-26
  Under The Limit (UndrLim) : Subsystem
  LKAInP_bsLKAInPInfo : Outport
  wires:
  LKAInP_bsInInfoSyn/1 -> TTLC Calculation (TTLCCalc)/3(bsInfo), Previewed Deviation Calculation (PrDvt)/2(PrvwDvt_bsInInfoSyn), Previewed Heading Angle Calculation (PrHdAg)/1(PrHdAg_bsInInfoSyn), Previewed Curvature Calculation (PrCrvt)/1(PrvwCrvt_bsInInfoSyn), Deviation Calculation (Dvt)/1(Dvt_bsInInfoSyn), Heading Angle Calculation (HdAg)/1(HdAg_bsInInfoSyn), Curvature Calculation (Crvt)/1(PrvwCrvt_bsInInfoSyn), Under The Limit (UndrLim)/1(UndrLim_bsInInfoSyn), Steering Wheel Position Calculation (SWAPosCal)/1(SWAPosCal_bsInInfoSyn), Lane Width Calculation (LW)/1(LW_bsInInfoSyn)
  Heading Angle Calculation (HdAg)/1(HdAg_bsHdAgInfo) -> Bus Creator2/5, TTLC Calculation (TTLCCalc)/5(In5)  "bsHdAgInfo"
  LKAInP_bsLLClb/1 -> Previewed Heading Angle Calculation (PrHdAg)/2(PrHdAg_bsLLClb), Under The Limit (UndrLim)/2(UndrLim_bsLLClb), Steering Wheel Position Calculation (SWAPosCal)/2(SWAPosCal_bsLLClb), Deviation Calculation (Dvt)/2(Dvt_bsLLClb), Previewed Curvature Calculation (PrCrvt)/2(PrvwCrvt_tiCrvtPrvwT_C), TTLC Calculation (TTLCCalc)/2(bsLLClb), Previewed Deviation Calculation (PrDvt)/1(PrdcDvt_bsLLClb)
  Previewed Heading Angle Calculation (PrHdAg)/1(PrHdAg_bsPrHdAgInfo) -> Bus Creator2/8  "bsPrHdAgInfo"
  TTLC Calculation (TTLCCalc)/1(TTLCCalc_bsTTLCInfo) -> Previewed Heading Angle Calculation (PrHdAg)/3(PrHdAg_bsTTLCInfo), Bus Creator2/10  "bsTTLCInfo"
  Lane Width Calculation (LW)/1(LW_LaneWidth) -> Bus Creator2/1  "LaneWidth"
  Steering Wheel Position Calculation (SWAPosCal)/1(SWAPosCal) -> Bus Creator2/2  "phiSWAPos"
  Under The Limit (UndrLim)/1(UndrLim_bsUndrLimInfo) -> Bus Creator2/3  "bsUndrLimInfo"
  Deviation Calculation (Dvt)/1(Dvt_bsDvtInfo) -> TTLC Calculation (TTLCCalc)/1(bsDvtInfo), Bus Creator2/6  "bsDvtInfo"
  Curvature Calculation (Crvt)/1(Crvt_bsCrvtInfo) -> Bus Creator2/4  "bsCrvtInfo"
  Previewed Deviation Calculation (PrDvt)/1(PrvwDvt_bsPrvwDvtInfo) -> Bus Creator2/9  "bsPrDvtInfo"
  Previewed Curvature Calculation (PrCrvt)/1(PrvwCrvt_bsPrvwCrvtInfo) -> Bus Creator2/7, TTLC Calculation (TTLCCalc)/4(In4)  "bsPrCrvtInfo"
  Bus Creator2/1 -> LKAInP_bsLKAInPInfo/1
  In3/1 -> Delay/1
  Delay/1 -> Previewed Curvature Calculation (PrCrvt)/3(PrvwCrvt_stLKAActvFlg)

== system MIL4L3_SW6_V1_20220211/CarMaker/VehicleControl/Function/LKA/LKAS1/LL/LLOn/LL State Determination (LLStateDet) ==
  LLStateDet_bsInInfoSyn : Inport
  LLStateDet_bsLKAInPInfo : Inport  Port=2
  LLStateDet_bsLLClb : Inport  Port=3
  LLStateDet_stExitFlg : Inport  Port=4
  LLStateDet_SignalFault : Inport  Port=5
  Bus Creator : BusCreator  Inputs=3
  Delay : Delay  DelayLength=1
  Delay1 : Delay  DelayLength=1
  LDW_State_Machine : Stateflow chart  Description=|  TreatAsAtomicUnit=on
      | Block Name: LDW State Machine
      | Ab.: LDWSM
      | No.: 1.1.2.0
      | Rev: 0.0.1
      | Update Date: 19-3-26
      settings: RTWSystemCode=Nonreusable function
  LKA_State_Machine : Stateflow chart  Description=|  TreatAsAtomicUnit=on
      | Block Name: LKA State Machine
      | Ab.: LKASM
      | No.: 1.1.3.0
      | Rev: 0.0.1
      | Update Date: 19-3-26
      settings: RTWSystemCode=Nonreusable function
  LL State Machine Conditions (LLSMCon) : Subsystem
  LLStateDet_bsLLState : Outport
  LLStateDet_stLDWActvFlg : Outport  Port=2
  LLStateDet_stLKAActvFlg : Outport  Port=3
  Disable_Reason : Outport  Port=4
  tag scope: LDW_State_Mon=global, LKA_State_Mon=global
  wires:
  LL State Machine Conditions (LLSMCon)/2(LLSMCon_stLDWEnaCSyn) -> LDW_State_Machine/2(LDWSM_stEnaCSyn)
  LL State Machine Conditions (LLSMCon)/3(LLSMCon_stLDWDisblCSyn) -> LDW_State_Machine/3(LDWSM_stDisblCSyn)
  LL State Machine Conditions (LLSMCon)/4(LLSMCon_stLDWActvCSyn) -> LDW_State_Machine/4(LDWSM_stActvCSyn)
  LL State Machine Conditions (LLSMCon)/5(LLSMCon_stLDWDeactvCSyn) -> LDW_State_Machine/5(LDWSM_stDeactvCSyn)
  LL State Machine Conditions (LLSMCon)/1(LLSMCon_stDACMode) -> Bus Creator/2, LKA_State_Machine/1(LKASM_stLMCMode), LDW_State_Machine/1(LDWSM_stLMCMode)  "DACMode"
  LDW_State_Machine/1(LDWSM_stLDWActvFlg) -> LLStateDet_stLDWActvFlg/1
  LKA_State_Machine/1(LKASM_stLKAActvFlg) -> LLStateDet_stLKAActvFlg/1
  Delay1/1 -> LL State Machine Conditions (LLSMCon)/4(LLSMCon_bsLLState)
  Bus Creator/1 -> LLStateDet_bsLLState/1, Delay1/1  "LLState"
  LKA_State_Machine/2(LKASM_stLKAState) -> [LKA_State_Mon], Bus Creator/3  "LKA_State"
  LDW_State_Machine/2(LDWSM_stLDWState) -> [LDW_State_Mon], Bus Creator/1  "LDW_State"
  LL State Machine Conditions (LLSMCon)/6(LLSMCon_stLDWFaultCSyn) -> LDW_State_Machine/6(LDWSM_stFaultCSyn)
  LL State Machine Conditions (LLSMCon)/7(LLSMCon_stLKAEnaCSyn) -> LKA_State_Machine/2(LKASM_stEnaCSyn)
  LL State Machine Conditions (LLSMCon)/8(LLSMCon_stLKADisblCSyn) -> LKA_State_Machine/3(LKASM_stDisblCSyn)
  LL State Machine Conditions (LLSMCon)/9(LLSMCon_stLKAActvCSyn) -> LKA_State_Machine/4(LKASM_stActvCSyn)
  LL State Machine Conditions (LLSMCon)/10(LLSMCon_stLKADeactvCSyn) -> LKA_State_Machine/5(LKASM_stDeactvCSyn)
  LL State Machine Conditions (LLSMCon)/11(LLSMCon_stLKAFaultCSyn) -> LKA_State_Machine/6(LKASM_stFaultCSyn)
  LLStateDet_bsInInfoSyn/1 -> LL State Machine Conditions (LLSMCon)/1(LLSMCon_bsInInfoSyn)
  LLStateDet_bsLKAInPInfo/1 -> LL State Machine Conditions (LLSMCon)/2(LLSMCon_bsLKAInPInfo)
  LLStateDet_stExitFlg/1 -> Delay/1
  LLStateDet_bsLLClb/1 -> LL State Machine Conditions (LLSMCon)/3(LLSMCon_bsLLClb)
  Delay/1 -> LL State Machine Conditions (LLSMCon)/5(LLSMCon_stExitFlg)
  LLStateDet_SignalFault/1 -> LL State Machine Conditions (LLSMCon)/6(LLSMCon_bsSignalFault)
  LL State Machine Conditions (LLSMCon)/12(Disable_Reason) -> Disable_Reason/1

== system MIL4L3_SW6_V1_20220211/CarMaker/VehicleControl/Function/LKA/LKAS1/LL/LLOn/LL_Mon ==
  Disable_Reason : Inport
  LKAMon : Inport  Port=2
  Bus : BusCreator  Inputs=4
  BusInP : BusCreator  Inputs=2
  BusState : BusCreator  Inputs=2
  LLMon : Outport
  wires:
  [InPMon] -> Bus/1
  [StateMon] -> Bus/2
  LKAMon/1 -> Bus/3
  Bus/1 -> LLMon/1  "LLMon"
  [LFTTTLC_Mon] -> BusInP/1  "LFTTTLC_Mon"
  [RGTTTLC_Mon] -> BusInP/2  "RGTTTLC_Mon"
  [LDW_State_Mon] -> BusState/1  "LDW_State_Mon"
  [LKA_State_Mon] -> BusState/2  "LKA_State_Mon"
  BusInP/1 -> [InPMon]  "InPMon"
  BusState/1 -> [StateMon]  "StateMon"
  Disable_Reason/1 -> Bus/4  "Disable_Reason"
